simulink model "diab_for_stat3__2016a_d1type_L1"  (R2016a)
settings: Solver=VariableStepAuto  StartTime=0.0  StopTime=24*7  RelTol=1e-6
undefined symbols (not defined in the file): normpdf
libraries: simulink x13
settings Model: Creator=Alex  LastModifiedBy=Alex
settings SolverCC: ZeroCrossAlgorithm=Adaptive

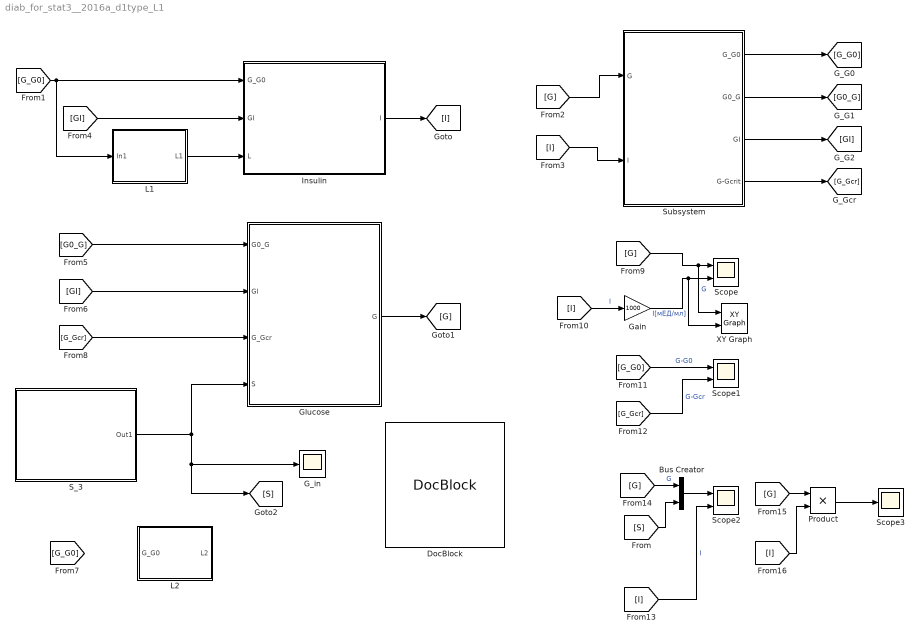
== system diab_for_stat3__2016a_d1type_L1 ==
  Bus Creator : BusCreator  Inputs=2
  DocBlock : simulink/Model-Wide Utilities/DocBlock  DocumentType=Text
      content=|
      | Моделируется диабет первого типа
      |
      | Организм пациента продуцирует инсулин в меньшем, чем требуется количестве
      | при этом инсулин "нормального качества", то есть элиминирует глюкозу нормальным
      | образом
      |
      | Моделируется снижением коэффициента альфа в 5 раз,
      | уровень глюкозы (норма) - 6.4,
      | уровень элиминации глюкозы почками - 14
      |
      | Подключена система управления с пропорциональной уровню глюкозы подачей
      | инсулина (система L1)
  G_in : Scope
  Gain : Gain  Gain=1000
  Glucose : Subsystem
  Insulin : Subsystem
  L1 : Subsystem
  "L2 " : Subsystem
  Product : Product
  S_3 : Subsystem
  Scope : Scope  NumInputPorts=2
  Scope1 : Scope  NumInputPorts=2
  Scope2 : Scope  NumInputPorts=2
  Scope3 : Scope
  Subsystem : Subsystem
  XY Graph : simulink/Sinks/XY Graph  xmin=2  xmax=12  ymin=-1  ymax=150  st=-1
  wires:
  [I] -> Gain/1  "I"
  [G] -> XY Graph/1, Scope/1  "G"
  [G_G0] -> Scope1/1  "G-G0"
  [G_Gcr] -> Scope1/2  "G-Gcr"
  [G] -> Subsystem/1(G)
  [I] -> Subsystem/2(I)
  Subsystem/1(G_G0) -> [G_G0]
  Subsystem/2(G0_G) -> [G0_G]
  Subsystem/3(GI) -> [GI]
  Subsystem/4(G-Gcrit) -> [G_Gcr]
  [G_G0] -> L1/1(In1), Insulin/1(G_G0)
  [GI] -> Insulin/2(GI)
  Insulin/1(I) -> [I]
  [G0_G] -> Glucose/1(G0_G)
  [GI] -> Glucose/2(GI)
  [G_Gcr] -> Glucose/3(G_Gcr)
  S_3/1(Out1) -> Glucose/4(S), [S], G_in/1
  Glucose/1(G) -> [G]
  L1/1(L1) -> Insulin/3(L)
  [I] -> Scope2/2  "I"
  [G] -> Bus Creator/1  "G"
  [S] -> Bus Creator/2
  Bus Creator/1 -> Scope2/1
  [G] -> Product/1
  [I] -> Product/2
  Product/1 -> Scope3/1
  Gain/1 -> XY Graph/2, Scope/2  "I[мЕД/мл]"

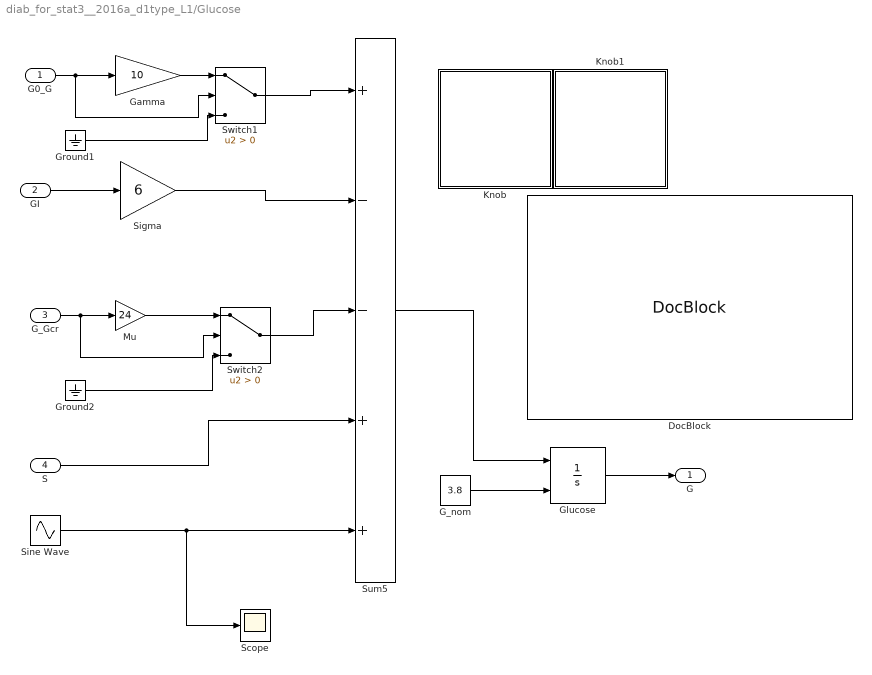
== system diab_for_stat3__2016a_d1type_L1/Glucose ==
  G0_G : Inport
  GI : Inport  Port=2
  G_Gcr : Inport  Port=3
  S : Inport  Port=4
  DocBlock : simulink/Model-Wide Utilities/DocBlock  DocumentType=Text
      content=|
      | Моделируется уровень концентрации глюкозы
      |
      | Глюкоза поступает из организма, если ее уровень ниже номинального G0
      | Реализована функция Хэвисайда на управляемом переключателе
      | Управляющий сигнал - G0-G, он положителен, если уровень глюкозы мал
      | Ситуация может возникнуть, например, при выбросе адреналина,
      | в модели, в том числе,  играет роль страховки от нефизичных результатов
      | с отрицательными концентрациями глюкозы
      |
      | Глюкоза элиминируется пропорционально концентрациям G и I как произведения
      | с коэффициентом Sigma
      |
      | Глюкоза элиминируется с мочой почками при превышении критического уровня
      | G-Gcrit>0 с коэффициентом Mu. Помимо прочего, включена в модель для
      | контроля концентрации глюкозы "сверху"
      |
      | Вход S моделирует экзогенное поступление глюкозы. Моделируется через функцию
      | нормального распределения. Математическое ожидание - время максимальной
      | онцентрации глюкозы, стандартное отклонение (плюс-минус 2 сигма - не путать
      | с коэффициентом сигма системы ДУ) - общее время поступления глюкозы.
      |
      | Глюкоза задается концентрацией, поэтому за 1 поступление всегда будет
      | получено 1, а общее количество полученной глюкозы (в концентрации)
      | задается параметром величины - константы, на которую домножается функция
      | нормального распределения (см. комментарий к блоку).
      |
      | Синусоида моделирует суточные колебания уровня глюкозы (утром выше, чем днем.
      | Включено с прицелом на модификацию модели.
  G_nom : Constant  Value=3.8
  Gamma : Gain  Gain=10
  Glucose : Integrator  InitialConditionSource=external
  Ground1 : Ground
  Ground2 : Ground
  Knob : Subsystem  DialogController=hmiCreateDDGDialog  IsWebBlock=on  mask(MWDashboardBlock){webBlockId=72e3f933-df98-437f-99fb-e333308aeccf, webBlockType=continuousknob, ShowInLibBrowser=on, ShowInitialText=on, HMISrcModelName=diab_for_stat3__2016a_d1type_L1}
      mask prompts: webBlockId "WebBlock Id"; webBlockType "WebBlock Type"; HMISrcModelName "Source Model"
      mask Help: helpview([docroot '/mapfiles/simulink.map'], 'hmi_knob')
      mask Display:
      | if strcmp(get_param(bdroot(gcb),'BlockDiagramType'), 'library')
      |     image([(matlabroot) '/toolbox/simulink/hmi/icons/ContinuousKnob.png']);
      | end
  Knob1 : Subsystem  DialogController=hmiCreateDDGDialog  IsWebBlock=on  mask(MWDashboardBlock){webBlockId=069f1754-ba14-4630-9e25-2dd9c45df99b, webBlockType=continuousknob, ShowInLibBrowser=on, ShowInitialText=on, HMISrcModelName=diab_for_stat3__2016a_d1type_L1}
      mask prompts: webBlockId "WebBlock Id"; webBlockType "WebBlock Type"; HMISrcModelName "Source Model"
      mask Help: helpview([docroot '/mapfiles/simulink.map'], 'hmi_knob')
      mask Display:
      | if strcmp(get_param(bdroot(gcb),'BlockDiagramType'), 'library')
      |     image([(matlabroot) '/toolbox/simulink/hmi/icons/ContinuousKnob.png']);
      | end
  Mu : Gain  Gain=24
  Scope : Scope
  Sigma : Gain  Gain=6
  Sine Wave : Sin  Amplitude=0.6  Frequency=2*pi/24  Phase=-0.4  SampleTime=0
  Sum5 : Sum  Inputs=+--++
  Switch1 : Switch  Criteria=u2 > Threshold
  Switch2 : Switch  Criteria=u2 > Threshold
  G : Outport
  wires:
  Ground1/1 -> Switch1/3
  Gamma/1 -> Switch1/1
  G_Gcr/1 -> Switch2/2, Mu/1
  G_nom/1 -> Glucose/2
  Mu/1 -> Switch2/1
  Switch2/1 -> Sum5/3
  Ground2/1 -> Switch2/3
  Switch1/1 -> Sum5/1
  G0_G/1 -> Switch1/2, Gamma/1
  Sum5/1 -> Glucose/1
  Glucose/1 -> G/1
  GI/1 -> Sigma/1
  Sigma/1 -> Sum5/2
  S/1 -> Sum5/4
  Sine Wave/1 -> Scope/1, Sum5/5

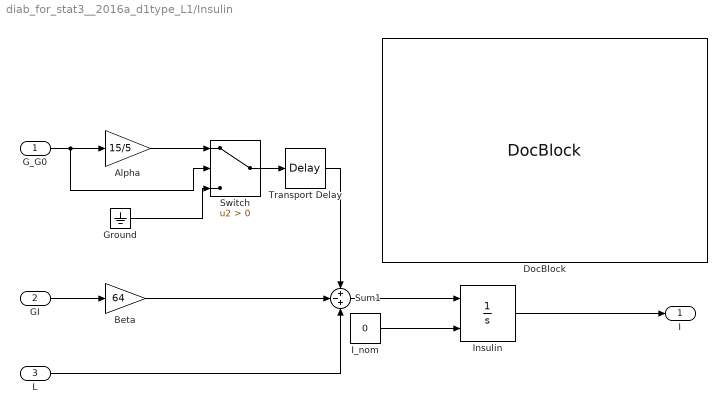
== system diab_for_stat3__2016a_d1type_L1/Insulin ==
  G_G0 : Inport
  GI : Inport  Port=2
  L : Inport  Port=3
  Alpha : Gain  Gain=15/5
  Beta : Gain  Gain=64
  DocBlock : simulink/Model-Wide Utilities/DocBlock  DocumentType=Text
      content=|
      | Блок, описывающий генерацию и элиминацию инсулина.
      | Рассматриватеся только активный инсулин
      | Инсулин вырабатывается при превышении концентрации глюкозы выше ее номинального
      | уровня G0 (вход G-G0)
      | Для этого реализована функция Хэвисайда через выключатель
      |
      | При положительном сигнале G-G0 вырабатывается инсулин пропорционально
      | указанному сигналу с коэффициентом Alfa
      | имеется возможность задать время задержки генерации инсулина по отношению
      | ко времени превышения номинального уровня
      |
      | Инсулин элиминируется с коэффициентом Beta, пропорционально произведению
      | концентраций G и I
      |
      | Вход L предназначен для моделирования подачи инсулина, например -
      | инсулиновой помпой или иначе
  Ground : Ground
  I_nom : Constant  Value=0
  Insulin : Integrator  InitialConditionSource=external
  Sum1 : Sum  Inputs=+-+
  Switch : Switch  Criteria=u2 > Threshold
  Transport Delay : TransportDelay  DelayTime=8/60
  I : Outport
  wires:
  I_nom/1 -> Insulin/2
  Beta/1 -> Sum1/2
  Alpha/1 -> Switch/1
  Sum1/1 -> Insulin/1
  Ground/1 -> Switch/3
  G_G0/1 -> Switch/2, Alpha/1
  GI/1 -> Beta/1
  Switch/1 -> Transport Delay/1
  L/1 -> Sum1/3
  Transport Delay/1 -> Sum1/1
  Insulin/1 -> I/1

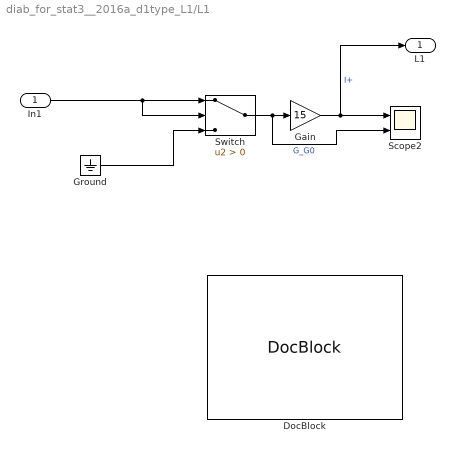
== system diab_for_stat3__2016a_d1type_L1/L1 ==
  In1 : Inport
  DocBlock : simulink/Model-Wide Utilities/DocBlock  DocumentType=Text
      content=|
      | Моделируется подача инсулина с переменной концентрацией
      | Концентрация определяется уровнем превышения концентрации глюкозы
      | относительно номинального G0
      | Подача включается при условии, что концентрация глюкозы превышает номинальную
      | на некоторую величину (может быть нулем, но как правило - величина,
      | большая нуля.
      | Уровень включения регулируется порогом управляемого выключателя, например
      | если G0 = 3.8
      | порог выключателя - 3
      | то подача инсулина произойдет при концентрации глюкозы 3.8+3=6.8
      |
      | Необходжимо согласовывать единицы измерения!!!
  Gain : Gain  Gain=15
  Ground : Ground
  Scope2 : Scope  NumInputPorts=2
  Switch : Switch  Criteria=u2 > Threshold
  L1 : Outport
  wires:
  Switch/1 -> Scope2/2, Gain/1  "G_G0"
  In1/1 -> Switch/2, Switch/1
  Gain/1 -> L1/1, Scope2/1  "I+"
  Ground/1 -> Switch/3

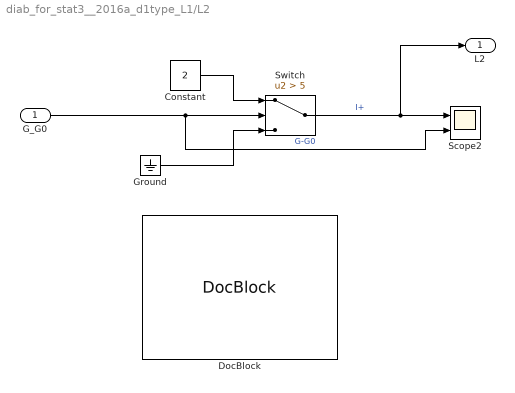
== system diab_for_stat3__2016a_d1type_L1/L2  ==
  G_G0 : Inport
  Constant : Constant  Value=2
  DocBlock : simulink/Model-Wide Utilities/DocBlock  DocumentType=Text
      content=|
      | Моделируется подача инсулина с постоянной концентрацией
      | Концентрация задана константой
      | Подача включается при условии, что концентрация глюкозы превышает номинальную
      | на некоторую величину (может быть нулем, но как правило - величина,
      | большая нуля.
      | Уровень включения регулируется порогом управляемого выключателя, например
      | если G0 = 3.8
      | порог выключателя - 3
      | то подача инсулина произойдет при концентрации глюкозы 3.8+3=6.8
      |
      | Необходжимо согласовывать единицы измерения!!!
  Ground : Ground
  Scope2 : Scope  NumInputPorts=2
  Switch : Switch  Criteria=u2 > Threshold  Threshold=5
  L2 : Outport
  wires:
  Constant/1 -> Switch/1
  Switch/1 -> L2/1, Scope2/1  "I+"
  G_G0/1 -> Switch/2, Scope2/2  "G-G0"
  Ground/1 -> Switch/3

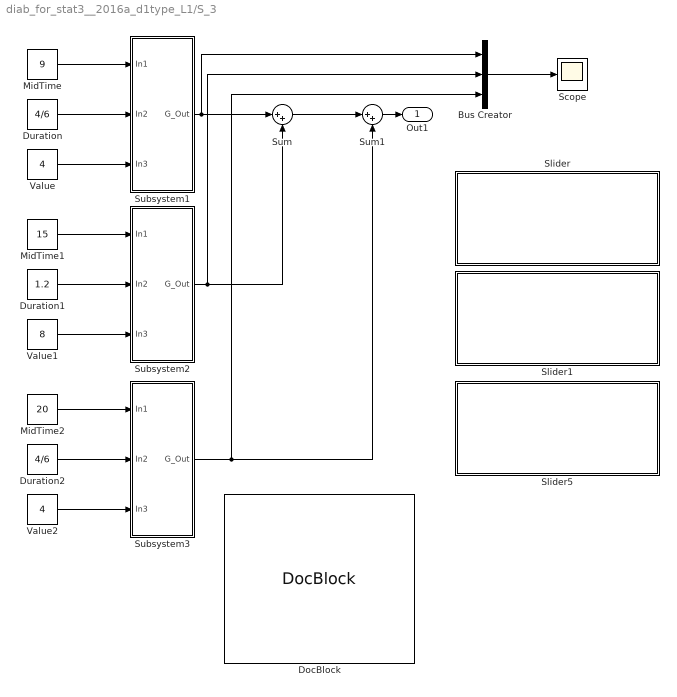
== system diab_for_stat3__2016a_d1type_L1/S_3 ==
  Bus Creator : BusCreator  Inputs=3
  DocBlock : simulink/Model-Wide Utilities/DocBlock  DocumentType=Text
      content=|
      | Модель трехкратного экзогенного поступления глюкозы
      |
      | Можно рассматривать как модуль подачи фиксированного объема глюкозы
      | в определенное время три раза в день
      |
      | Можно рассматривать как результат приема пищи и выработки глюкозы вседствие
      | этого.
      |
      | Блоки позволяют варьировать время максимальной концентрации глюкозы,
      | общее время ее подачи (исходя из того, что кривая поступления моделируется
      | кривой Гауса, причем используется правило 4 сигма.
      | Можно считать, что подача начинается за 2сигма (половину общего времени
      | подачи глюкозы)и заканчивается через 2сигма после, а концентрация подчиняется
      | закону нормального распределения.
      |
      | За это время будет подано Value глюкозы (выраженное через  концентрацию) или
      | строго говоря 95% указанной величины
      |
      | Моделируется трехразовая подача глюкозы (питание завтрак-обед-ужин)
      | Объем глюкозы задан в соотношении 1/4-1/2-1/4 соответственно.
      | Время поступления (расчетное время максимальной концентрации глюкозы)
      | 9-15-20 часов соответственно.
  Duration : Constant  Value=4/6
  Duration1 : Constant  Value=1.2
  Duration2 : Constant  Value=4/6
  MidTime : Constant  Value=9
  MidTime1 : Constant  Value=15
  MidTime2 : Constant  Value=20
  Scope : Scope
  Slider : Subsystem  DialogController=hmiCreateDDGDialog  IsWebBlock=on  mask(MWDashboardBlock){webBlockId=f1176611-fab8-43e0-a0bb-fa81c9901513, webBlockType=slider, ShowInLibBrowser=on, ShowInitialText=on, HMISrcModelName=diab_for_stat3__2016a_d1type_L1}
      mask prompts: webBlockId "WebBlock Id"; webBlockType "WebBlock Type"; HMISrcModelName "Source Model"
      mask Help: helpview([docroot '/mapfiles/simulink.map'], 'hmi_slider')
      mask Display:
      | if strcmp(get_param(bdroot(gcb),'BlockDiagramType'), 'library')
      |     image([(matlabroot) '/toolbox/simulink/hmi/icons/Slider.png']);
      | end
  Slider1 : Subsystem  DialogController=hmiCreateDDGDialog  IsWebBlock=on  mask(MWDashboardBlock){webBlockId=823537b8-b9ab-4a06-9138-fbfa3de8e097, webBlockType=slider, ShowInLibBrowser=on, ShowInitialText=on, HMISrcModelName=diab_for_stat3__2016a_d1type_L1}
      mask prompts: webBlockId "WebBlock Id"; webBlockType "WebBlock Type"; HMISrcModelName "Source Model"
      mask Help: helpview([docroot '/mapfiles/simulink.map'], 'hmi_slider')
      mask Display:
      | if strcmp(get_param(bdroot(gcb),'BlockDiagramType'), 'library')
      |     image([(matlabroot) '/toolbox/simulink/hmi/icons/Slider.png']);
      | end
  Slider5 : Subsystem  DialogController=hmiCreateDDGDialog  IsWebBlock=on  mask(MWDashboardBlock){webBlockId=00a66d36-902f-4290-86fc-c4a990b459a4, webBlockType=slider, ShowInLibBrowser=on, ShowInitialText=on, HMISrcModelName=diab_for_stat3__2016a_d1type_L1}
      mask prompts: webBlockId "WebBlock Id"; webBlockType "WebBlock Type"; HMISrcModelName "Source Model"
      mask Help: helpview([docroot '/mapfiles/simulink.map'], 'hmi_slider')
      mask Display:
      | if strcmp(get_param(bdroot(gcb),'BlockDiagramType'), 'library')
      |     image([(matlabroot) '/toolbox/simulink/hmi/icons/Slider.png']);
      | end
  Subsystem1 : Subsystem
  Subsystem2 : Subsystem
  Subsystem3 : Subsystem
  Sum : Sum  Inputs=|++
  Sum1 : Sum  Inputs=|++
  Value : Constant  Value=4
  Value1 : Constant  Value=8
  Value2 : Constant  Value=4
  Out1 : Outport
  wires:
  Value2/1 -> Subsystem3/3(In3)
  Duration2/1 -> Subsystem3/2(In2)
  MidTime2/1 -> Subsystem3/1(In1)
  Duration/1 -> Subsystem1/2(In2)
  Value/1 -> Subsystem1/3(In3)
  Subsystem1/1(G_Out) -> Bus Creator/1, Sum/1
  Subsystem2/1(G_Out) -> Bus Creator/2, Sum/2
  MidTime/1 -> Subsystem1/1(In1)
  Sum/1 -> Sum1/1
  Value1/1 -> Subsystem2/3(In3)
  MidTime1/1 -> Subsystem2/1(In1)
  Duration1/1 -> Subsystem2/2(In2)
  Sum1/1 -> Out1/1
  Bus Creator/1 -> Scope/1
  Subsystem3/1(G_Out) -> Bus Creator/3, Sum1/2

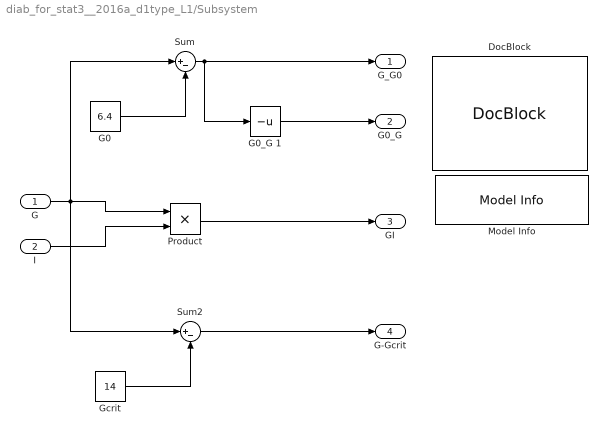
== system diab_for_stat3__2016a_d1type_L1/Subsystem ==
  G : Inport
  I : Inport  Port=2
  DocBlock : simulink/Model-Wide Utilities/DocBlock  DocumentType=Text  mask(DocBlock){}
      content=|
      | Блок устанавливает:
      | G0 - номинальный уровень глюкозы пациента
      | выше него - вырабатывается активный инсулин
      | ниже него - вырабатывается глюкоза, например - из печени
      | Gcrit - критический, выше которого происхожит элиминация глюкозы почками
      | GI - уровень концентрации глюкозы совместно с концентрацией активного инсулина
      | пропорционально этому произведению элиминируется глюкоза и инсулин
  G0 : Constant  Value=6.4
  G0_G 1 : UnaryMinus
  Gcrit : Constant  Value=14
  Model Info : simulink/Model-Wide Utilities/Model Info  Frame=on  DisplayStringWithTags=|  HorizontalTextAlignment=Center  LeftAlignmentValue=0.5  SourceBlockDiagram=diab_for_stat3__2016a_d1type_L1  TagMaxNumber=20
      | Model Info
      | %<Creator>
      | %<ModifiedDate>
      | %<Description>
  Product : Product
  Sum : Sum  Inputs=|+-
  Sum2 : Sum  Inputs=|+-
  G_G0 : Outport
  G0_G : Outport  Port=2
  GI : Outport  Port=3
  G-Gcrit : Outport  Port=4
  wires:
  G0/1 -> Sum/2
  Sum/1 -> G_G0/1, G0_G 1/1
  Gcrit/1 -> Sum2/2
  I/1 -> Product/2
  Sum2/1 -> G-Gcrit/1
  G/1 -> Sum2/1, Sum/1, Product/1
  G0_G 1/1 -> G0_G/1
  Product/1 -> GI/1

== system diab_for_stat3__2016a_d1type_L1/Glucose/Knob ==

== system diab_for_stat3__2016a_d1type_L1/Glucose/Knob1 ==

== system diab_for_stat3__2016a_d1type_L1/S_3/Slider ==

== system diab_for_stat3__2016a_d1type_L1/S_3/Slider1 ==

== system diab_for_stat3__2016a_d1type_L1/S_3/Slider5 ==

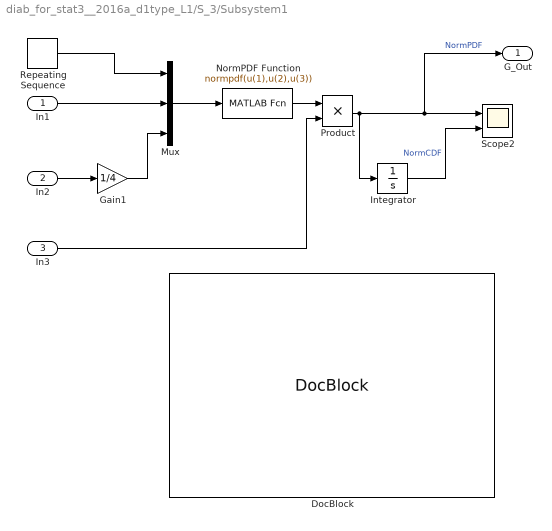
== system diab_for_stat3__2016a_d1type_L1/S_3/Subsystem1 ==
  In1 : Inport
  In2 : Inport  Port=2
  In3 : Inport  Port=3
  DocBlock : simulink/Model-Wide Utilities/DocBlock  DocumentType=Text
      content=|
      | модель подачи глюкозы (один прием)
      | "Пила" - нарастающий сигнал, эмулирует время (за 24 часа растет от 0 до 24)
      | Нужен для моделирования процессов, посторяющихся с интервалом в сутки
      |
      | in1 - время максимальной концентрации глюкозы - матожидание функции
      | нормального распределения
      | in2 - длительность приема, делим на 4 - получаем стандартное отклонение
      |
      | Функция Matlab - normpdf(u(1),u(2),u(3))
      | u(1) - время, u(2) - матожидание,  u(3) - стандартное отклонение
      | Чтобы их передать функции в правильном порядке - смешиваем данные в шине
      | (блок bus)
      |
      | Результат множим на коэффициент общего количества глюкозы in3
  Gain1 : Gain  Gain=1/4
  Integrator : Integrator
  Mux : Mux  Inputs=3
  NormPDF Function : MATLABFcn  MATLABFcn=normpdf(u(1),u(2),u(3))
  Product : Product
  Repeating Sequence : simulink/Sources/Repeating Sequence  rep_seq_t=[0 24]  rep_seq_y=[0 24]
  Scope2 : Scope  NumInputPorts=2
  G_Out : Outport
  wires:
  In2/1 -> Gain1/1
  Product/1 -> Integrator/1, G_Out/1, Scope2/1  "NormPDF"
  In1/1 -> Mux/2
  NormPDF Function/1 -> Product/1
  Integrator/1 -> Scope2/2  "NormCDF"
  Mux/1 -> NormPDF Function/1
  In3/1 -> Product/2
  Gain1/1 -> Mux/3
  Repeating Sequence/1 -> Mux/1

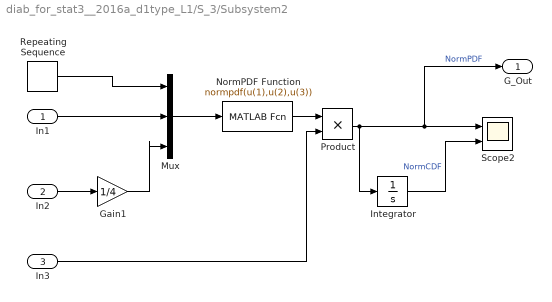
== system diab_for_stat3__2016a_d1type_L1/S_3/Subsystem2 ==
  In1 : Inport
  In2 : Inport  Port=2
  In3 : Inport  Port=3
  Gain1 : Gain  Gain=1/4
  Integrator : Integrator
  Mux : Mux  Inputs=3
  NormPDF Function : MATLABFcn  MATLABFcn=normpdf(u(1),u(2),u(3))
  Product : Product
  Repeating Sequence : simulink/Sources/Repeating Sequence  rep_seq_t=[0 24]  rep_seq_y=[0 24]
  Scope2 : Scope  NumInputPorts=2
  G_Out : Outport
  wires:
  In3/1 -> Product/2
  Mux/1 -> NormPDF Function/1
  Integrator/1 -> Scope2/2  "NormCDF"
  NormPDF Function/1 -> Product/1
  In1/1 -> Mux/2
  Repeating Sequence/1 -> Mux/1
  Gain1/1 -> Mux/3
  Product/1 -> Scope2/1, G_Out/1, Integrator/1  "NormPDF"
  In2/1 -> Gain1/1

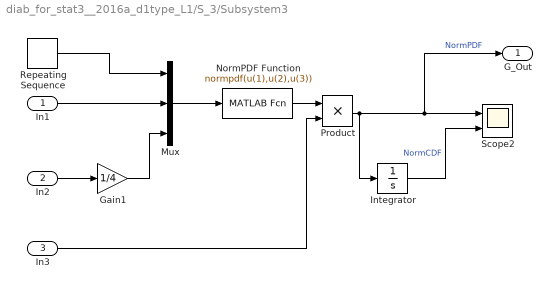
== system diab_for_stat3__2016a_d1type_L1/S_3/Subsystem3 ==
  In1 : Inport
  In2 : Inport  Port=2
  In3 : Inport  Port=3
  Gain1 : Gain  Gain=1/4
  Integrator : Integrator
  Mux : Mux  Inputs=3
  NormPDF Function : MATLABFcn  MATLABFcn=normpdf(u(1),u(2),u(3))
  Product : Product
  Repeating Sequence : simulink/Sources/Repeating Sequence  rep_seq_t=[0 24]  rep_seq_y=[0 24]
  Scope2 : Scope  NumInputPorts=2
  G_Out : Outport
  wires:
  In2/1 -> Gain1/1
  Product/1 -> Integrator/1, G_Out/1, Scope2/1  "NormPDF"
  Gain1/1 -> Mux/3
  In1/1 -> Mux/2
  NormPDF Function/1 -> Product/1
  Integrator/1 -> Scope2/2  "NormCDF"
  Mux/1 -> NormPDF Function/1
  In3/1 -> Product/2
  Repeating Sequence/1 -> Mux/1
